simulink model "EMG_System"  (R2022a)
settings: Solver=FixedStepAuto  StartTime=0.0  StopTime=30  FixedStep=0.001  RelTol=1e-3
undefined symbols (not defined in the file): fdesignblkfcn, gcbh, Serial_Port, Standard_Devices
libraries: sldrtlib x4, dspxfrm3 x2, dspstat3 x2
settings Model: Creator=Damian  LastModifiedBy=lunde
settings ModelReferenceCC: EnableRefExpFcnMdlSchedulingChecks=off
settings RTWCC: Description=Generic Real-Time Target

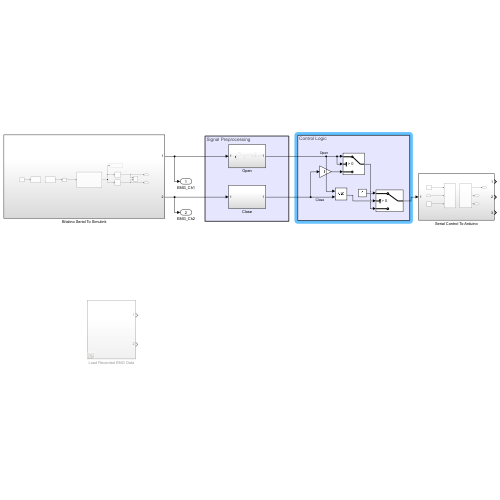
[thumbnail: Simulink's stored preview of the top-level diagram]
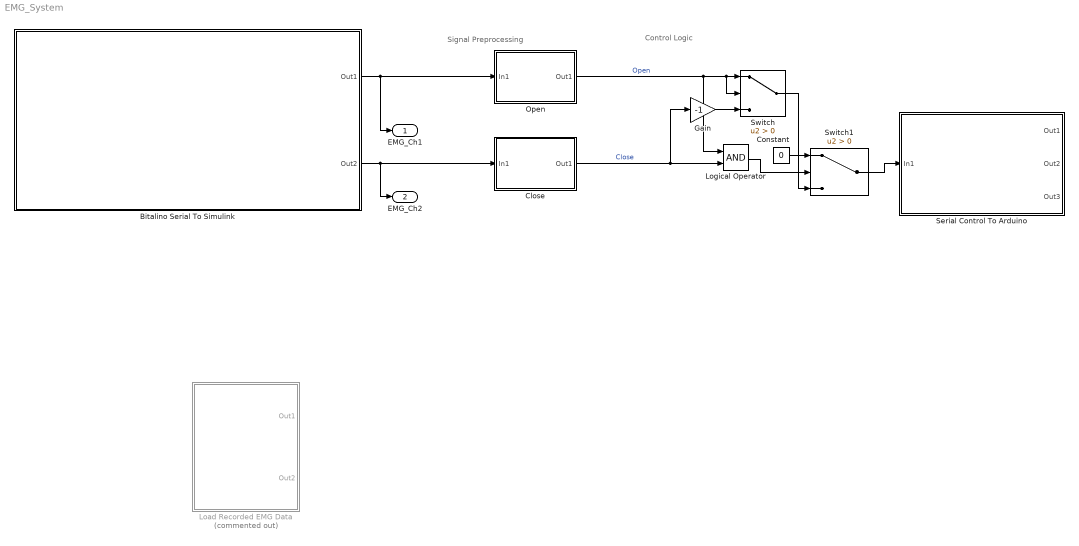
== system EMG_System ==
  note: Control Logic
  note: Signal Preprocessing
  Bitalino Serial To Simulink : Subsystem
  Close : Subsystem
  Constant : Constant  Value=0
  Gain : Gain  Gain=-1
  Load Recorded EMG Data : Subsystem  Commented=on
  Logical Operator : Logic  AllPortsSameDT=off  OutDataTypeStr=boolean
  Open : Subsystem
  Serial Control To Arduino : Subsystem
  Switch : Switch  Criteria=u2 > Threshold  SaturateOnIntegerOverflow=off  InputSameDT=off
  Switch1 : Switch  Criteria=u2 > Threshold  SaturateOnIntegerOverflow=off  InputSameDT=off
  EMG_Ch1 : Outport
  EMG_Ch2 : Outport  Port=2
  wires:
  Open/1(Out1) -> Switch/2, Switch/1, Logical Operator/1  "Open"
  Close/1(Out1) -> Logical Operator/2, Gain/1  "Close"
  Gain/1 -> Switch/3
  Logical Operator/1 -> Switch1/2
  Constant/1 -> Switch1/1
  Switch/1 -> Switch1/3
  Switch1/1 -> Serial Control To Arduino/1(In1)
  Bitalino Serial To Simulink/1(Out1) -> EMG_Ch1/1, Open/1(In1)
  Bitalino Serial To Simulink/2(Out2) -> EMG_Ch2/1, Close/1(In1)

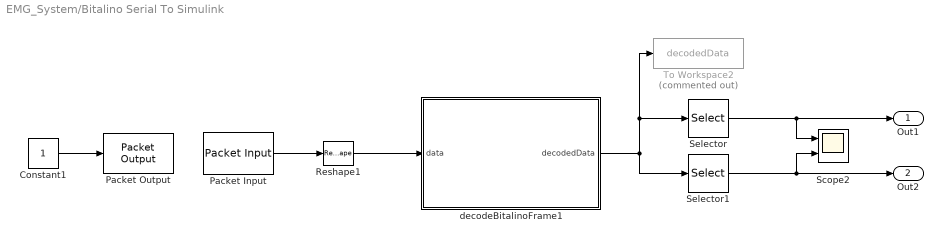
== system EMG_System/Bitalino Serial To Simulink ==
  Constant1 : Constant
  Packet Input : sldrtlib/Packet Input  SampleTime=0.001  MaxMissedTicks=10000  ShowMissedTicks=off  YieldWhenWaiting=on  DrvName=Standard_Devices/Serial_Port  DrvAddress=9  DrvOptions=[115200 8 0 0 0 0 0 0]  PacketSize=8  DataTypes='8*uint8'  ShowReady=off  ShowError=off  PacketID=1  ByteOrder=1  ShowTimestamp=off
      settings: AttributesFormatString=Serial Port [9]
  Packet Output : sldrtlib/Packet Output  SampleTime=0.001  MaxMissedTicks=10000  ShowMissedTicks=off  YieldWhenWaiting=on  DrvName=Standard_Devices/Serial_Port  DrvAddress=9  DrvOptions=[115200 8 0 0 0 0 0 0]  PacketSize=1  DataTypes='1*uint8'  ShowReady=off  ShowError=off  PacketID=1  ByteOrder=1  InitialValue=253  FinalValue=[]
      settings: AttributesFormatString=Serial Port [9]
  Reshape1 : Reshape  OutputDimensionality=Customize  OutputDimensions=[1,8]
  Scope2 : Scope  NumInputPorts=2
  Selector : Selector  InputPortWidth=2  IndexOptions=Index vector (dialog)  Indices=[1]  OutputSizes=1
  Selector1 : Selector  InputPortWidth=2  IndexOptions=Index vector (dialog)  Indices=[2]  OutputSizes=1
  To Workspace2 : ToWorkspace  Commented=on  VariableName=decodedData  SaveFormat=Timeseries  SampleTime=-1
  decodeBitalinoFrame1 : MATLAB Function  TreatAsAtomicUnit=on
  Out1 : Outport
  Out2 : Outport  Port=2
  wires:
  Selector/1 -> Out1/1, Scope2/1
  Selector1/1 -> Out2/1, Scope2/2
  Constant1/1 -> Packet Output/1
  Packet Input/1 -> Reshape1/1
  decodeBitalinoFrame1/1(decodedData) -> Selector1/1, To Workspace2/1, Selector/1
  Reshape1/1 -> decodeBitalinoFrame1/1(data)

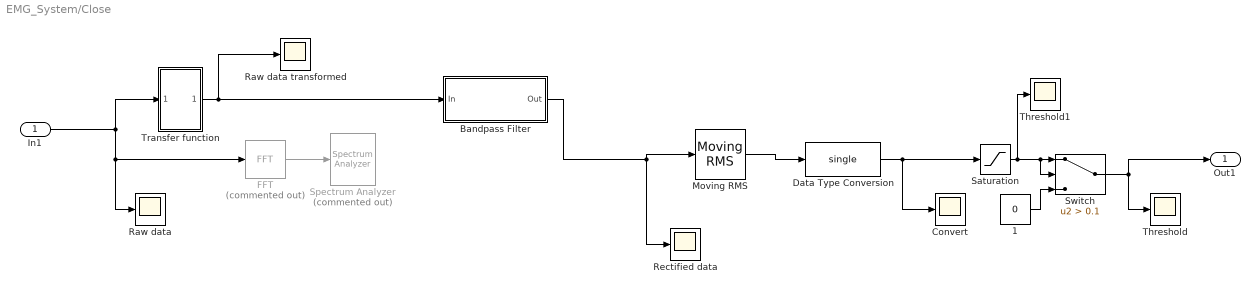
== system EMG_System/Close ==
  In1 : Inport
  1 : Constant  Value=0
  Bandpass Filter : Subsystem  DialogController=fdesignblkfcn  InitFcn=fdesignblkfcn(gcbh, {'InitFcn'});  mask(Bandpass Filter){}
      mask help: Design a bandpass filter
      settings: CopyFcn=fdesignblkfcn(gcbh, {'CopyFcn'});
      mask Help: helpview(mapfilelocation('dsp'), 'dspbandpassfilter');
      mask Display: disp('Bandpass');
  Convert : Scope
  Data Type Conversion : DataTypeConversion  OutMin=0  OutMax=1  OutDataTypeStr=single  RndMeth=Floor
  FFT : dspxfrm3/FFT  Commented=on  FFTImplementation=Auto  CompMethod=Table lookup  TableOpt=NEW  TableOptActive=Speed  BitRevOrder=off  Normalize=on  InheritFFTLength=on  FFTLength=64  WrapInput=on  roundingMode=Floor  overflowMode=off  firstCoeffDataTypeStr=Inherit: Same word length as input  firstCoeffLastDataTypeStr=Inherit: Same word length as input  outputMin=[]  outputMax=[]
  Moving RMS : dspstat3/Moving RMS  Method=Sliding window  ForgettingFactorPort=off  SpecifyWindowLength=on  WindowLength=100  ForgettingFactor=0.9  SimulateUsing=Code generation
      settings: SourceProductBaseCode=DS
  Raw data : Scope
  Raw data transformed : Scope
  Rectified data : Scope
  Saturation : Saturate  UpperLimit=0.8  LowerLimit=0.1
  Spectrum Analyzer : SpectrumAnalyzer  Commented=on
  Switch : Switch  Criteria=u2 > Threshold  Threshold=0.1  SaturateOnIntegerOverflow=off  InputSameDT=off
  Threshold : Scope
  Threshold1 : Scope
  Transfer function : Subsystem
  Out1 : Outport
  wires:
  Transfer function/1(Out1) -> Bandpass Filter/1(In), Raw data transformed/1
  FFT/1 -> Spectrum Analyzer/1
  1/1 -> Switch/3
  Bandpass Filter/1(Out) -> Moving RMS/1, Rectified data/1
  Moving RMS/1 -> Data Type Conversion/1
  Switch/1 -> Out1/1, Threshold/1
  In1/1 -> Transfer function/1(In1), Raw data/1, FFT/1
  Saturation/1 -> Threshold1/1, Switch/2, Switch/1
  Data Type Conversion/1 -> Saturation/1, Convert/1

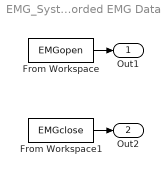
== system EMG_System/Load Recorded EMG Data ==
  From Workspace : FromWorkspace  VariableName=EMGopen
  From Workspace1 : FromWorkspace  VariableName=EMGclose
  Out1 : Outport
  Out2 : Outport  Port=2
  wires:
  From Workspace1/1 -> Out2/1
  From Workspace/1 -> Out1/1

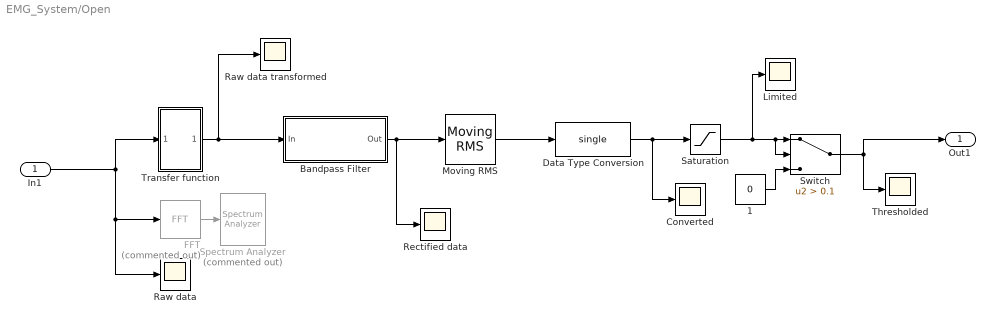
== system EMG_System/Open ==
  In1 : Inport
  1 : Constant  Value=0
  Bandpass Filter : Subsystem  DialogController=fdesignblkfcn  InitFcn=fdesignblkfcn(gcbh, {'InitFcn'});  mask(Bandpass Filter){}
      mask help: Design a bandpass filter
      settings: CopyFcn=fdesignblkfcn(gcbh, {'CopyFcn'});
      mask Help: helpview(mapfilelocation('dsp'), 'dspbandpassfilter');
      mask Display: disp('Bandpass');
  Converted : Scope
  Data Type Conversion : DataTypeConversion  OutMin=0  OutMax=1  OutDataTypeStr=single  RndMeth=Floor
  FFT : dspxfrm3/FFT  Commented=on  FFTImplementation=Auto  CompMethod=Table lookup  TableOpt=NEW  TableOptActive=Speed  BitRevOrder=off  Normalize=on  InheritFFTLength=on  FFTLength=64  WrapInput=on  roundingMode=Floor  overflowMode=off  firstCoeffDataTypeStr=Inherit: Same word length as input  firstCoeffLastDataTypeStr=Inherit: Same word length as input  outputMin=[]  outputMax=[]
  Limited : Scope
  Moving RMS : dspstat3/Moving RMS  Method=Sliding window  ForgettingFactorPort=off  SpecifyWindowLength=on  WindowLength=100  ForgettingFactor=0.9  SimulateUsing=Code generation
      settings: SourceProductBaseCode=DS
  Raw data : Scope
  Raw data transformed : Scope
  Rectified data : Scope
  Saturation : Saturate  UpperLimit=0.8  LowerLimit=0.1
  Spectrum Analyzer : SpectrumAnalyzer  Commented=on
  Switch : Switch  Criteria=u2 > Threshold  Threshold=0.1  SaturateOnIntegerOverflow=off  InputSameDT=off
  Thresholded : Scope
  Transfer function : Subsystem
  Out1 : Outport
  wires:
  Transfer function/1(Out1) -> Bandpass Filter/1(In), Raw data transformed/1
  FFT/1 -> Spectrum Analyzer/1
  1/1 -> Switch/3
  Bandpass Filter/1(Out) -> Moving RMS/1, Rectified data/1
  Moving RMS/1 -> Data Type Conversion/1
  Switch/1 -> Out1/1, Thresholded/1
  In1/1 -> Transfer function/1(In1), Raw data/1, FFT/1
  Saturation/1 -> Limited/1, Switch/2, Switch/1
  Data Type Conversion/1 -> Saturation/1, Converted/1

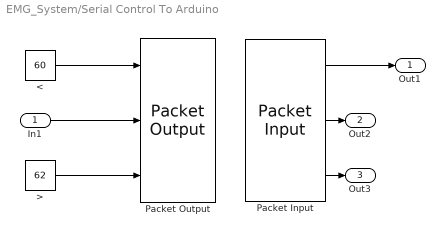
== system EMG_System/Serial Control To Arduino ==
  In1 : Inport  OutDataTypeStr=single  PortDimensions=1
  < : Constant  Value=60
  > : Constant  Value=62
  Packet Input : sldrtlib/Packet Input  SampleTime=0.1  MaxMissedTicks=1000  ShowMissedTicks=off  YieldWhenWaiting=off  DrvName=Standard_Devices/Serial_Port  DrvAddress=3  DrvOptions=[9600 8 0 0 0 0 0 0]  PacketSize=6  DataTypes={'1*single', '1*uint8', '1*uint8'}  ShowReady=off  ShowError=off  PacketID=1  ByteOrder=1  ShowTimestamp=off
      settings: AttributesFormatString=Serial Port [3]
  Packet Output : sldrtlib/Packet Output  SampleTime=0.1  MaxMissedTicks=1000  ShowMissedTicks=off  YieldWhenWaiting=off  DrvName=Standard_Devices/Serial_Port  DrvAddress=3  DrvOptions=[9600 8 0 0 0 0 0 0]  PacketSize=6  DataTypes={'1*uint8', '1*single', '1*uint8'}  ShowReady=off  ShowError=off  PacketID=1  ByteOrder=1  InitialValue=[]  FinalValue=[]
      settings: AttributesFormatString=Serial Port [3]
  Out1 : Outport
  Out2 : Outport  Port=2
  Out3 : Outport  Port=3
  wires:
  >/1 -> Packet Output/3
  In1/1 -> Packet Output/2
  </1 -> Packet Output/1
  Packet Input/2 -> Out2/1
  Packet Input/3 -> Out3/1
  Packet Input/1 -> Out1/1

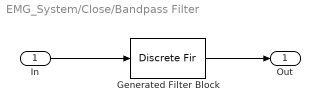
== system EMG_System/Close/Bandpass Filter ==
  In : Inport
  Generated Filter Block : DiscreteFir  Tag=BlockMethodSubSystem  Coefficients=[-0.000198473586190418182 0.00534852252952493484 0.0153234095334107579 0.0178570667191146684 0.00682248801041550508 -0.00274870515317482194 0.0030891279978422885 0.0111979036988692337 0.00456245530764537791 -0.0042151661328777134 0.00243546387977701222 0.00943183747086404935 -0.00146403536066665998 -0.011084600828395838 -0.00059029452559431156 0.00547540465791776249 -0.0119371461871073409 -0.0215599836706455474 -0.00473015163609309848 -0.000830348429932785187 -0.0270963317844445002 -0.034209054098530034 -0.00755561394207852031 -0.00849262478015036168 -0.0471568823138692056 -0.0469015880042323238 -0.00421271941163124924 -0.0158506365642964719 -0.0755462338263607064 -0.0571919323183570777 0.0195397096648971362 -0.0211950204421756522 -0.145410009473957602 -0.0629799708976308825 0.274125237654004761 0.476886321904536448 0.274125237654004761 -0.0629799708976308825 -0.145410009473957602 -0.0211950204421756522 0.0195397096648971362 -0.0571919323183570777 -0.0755462338263607064 -0.0158506365642964719 -0.00421271941163124924 -0.0469015880042323238 -0.0471568823138692056 -0.00849262478015036168 -0.00755561394207852031 -0.034209054098530034 -0.0270963317844445002 -0.000830348429932785187 -0.00473015163609309848 -0.0215599836706455474 -0.0119371461871073409 0.00547540465791776249 -0.00059029452559431156 -0.011084600828395838 -0.00146403536066665998 0.00943183747086404935 0.00243546387977701222 -0.0042151661328777134 0.00456245530764537791 0.0111979036988692337 0.0030891279978422885 -0.00274870515317482194 0.00682248801041550508 0.0178570667191146684 0.0153234095334107579 0.00534852252952493484 -0.000198473586190418182]  InputProcessing=Columns as channels (frame based)
  Out : Outport  VectorParamsAs1DForOutWhenUnconnected=off
  wires:
  In/1 -> Generated Filter Block/1
  Generated Filter Block/1 -> Out/1

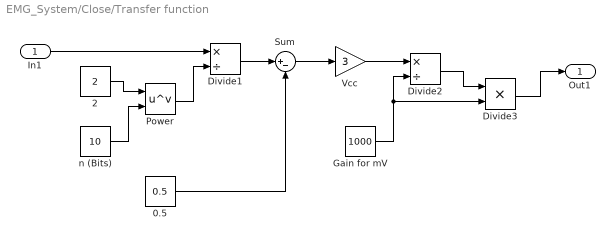
== system EMG_System/Close/Transfer function ==
  In1 : Inport
  0.5 : Constant  Value=0.5
  2 : Constant  Value=2
  Divide1 : Product  Inputs=*/
  Divide2 : Product  Inputs=*/
  Divide3 : Product  Inputs=**
  Gain for mV : Constant  Value=1000
  Power : Math  Operator=pow
  Sum : Sum  Inputs=|+-
  Vcc : Gain  Gain=3
  n (Bits) : Constant  Value=10
  Out1 : Outport
  wires:
  n (Bits)/1 -> Power/2
  In1/1 -> Divide1/1
  0.5/1 -> Sum/2
  Gain for mV/1 -> Divide3/2, Divide2/2
  Vcc/1 -> Divide2/1
  2/1 -> Power/1
  Power/1 -> Divide1/2
  Divide2/1 -> Divide3/1
  Divide3/1 -> Out1/1
  Divide1/1 -> Sum/1
  Sum/1 -> Vcc/1

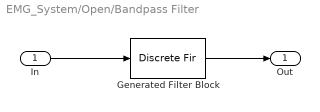
== system EMG_System/Open/Bandpass Filter ==
  In : Inport
  Generated Filter Block : DiscreteFir  Tag=BlockMethodSubSystem  Coefficients=[-0.000198473586190418182 0.00534852252952493484 0.0153234095334107579 0.0178570667191146684 0.00682248801041550508 -0.00274870515317482194 0.0030891279978422885 0.0111979036988692337 0.00456245530764537791 -0.0042151661328777134 0.00243546387977701222 0.00943183747086404935 -0.00146403536066665998 -0.011084600828395838 -0.00059029452559431156 0.00547540465791776249 -0.0119371461871073409 -0.0215599836706455474 -0.00473015163609309848 -0.000830348429932785187 -0.0270963317844445002 -0.034209054098530034 -0.00755561394207852031 -0.00849262478015036168 -0.0471568823138692056 -0.0469015880042323238 -0.00421271941163124924 -0.0158506365642964719 -0.0755462338263607064 -0.0571919323183570777 0.0195397096648971362 -0.0211950204421756522 -0.145410009473957602 -0.0629799708976308825 0.274125237654004761 0.476886321904536448 0.274125237654004761 -0.0629799708976308825 -0.145410009473957602 -0.0211950204421756522 0.0195397096648971362 -0.0571919323183570777 -0.0755462338263607064 -0.0158506365642964719 -0.00421271941163124924 -0.0469015880042323238 -0.0471568823138692056 -0.00849262478015036168 -0.00755561394207852031 -0.034209054098530034 -0.0270963317844445002 -0.000830348429932785187 -0.00473015163609309848 -0.0215599836706455474 -0.0119371461871073409 0.00547540465791776249 -0.00059029452559431156 -0.011084600828395838 -0.00146403536066665998 0.00943183747086404935 0.00243546387977701222 -0.0042151661328777134 0.00456245530764537791 0.0111979036988692337 0.0030891279978422885 -0.00274870515317482194 0.00682248801041550508 0.0178570667191146684 0.0153234095334107579 0.00534852252952493484 -0.000198473586190418182]  InputProcessing=Columns as channels (frame based)
  Out : Outport  VectorParamsAs1DForOutWhenUnconnected=off
  wires:
  In/1 -> Generated Filter Block/1
  Generated Filter Block/1 -> Out/1

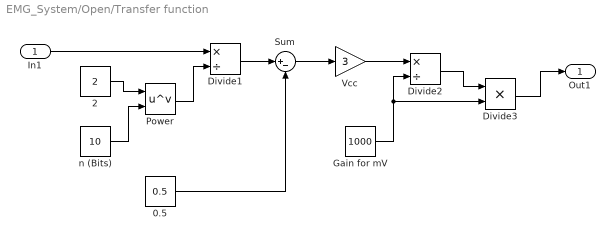
== system EMG_System/Open/Transfer function ==
  In1 : Inport
  0.5 : Constant  Value=0.5
  2 : Constant  Value=2
  Divide1 : Product  Inputs=*/
  Divide2 : Product  Inputs=*/
  Divide3 : Product  Inputs=**
  Gain for mV : Constant  Value=1000
  Power : Math  Operator=pow
  Sum : Sum  Inputs=|+-
  Vcc : Gain  Gain=3
  n (Bits) : Constant  Value=10
  Out1 : Outport
  wires:
  n (Bits)/1 -> Power/2
  In1/1 -> Divide1/1
  0.5/1 -> Sum/2
  Gain for mV/1 -> Divide3/2, Divide2/2
  Vcc/1 -> Divide2/1
  2/1 -> Power/1
  Power/1 -> Divide1/2
  Divide2/1 -> Divide3/1
  Divide3/1 -> Out1/1
  Divide1/1 -> Sum/1
  Sum/1 -> Vcc/1

== matlab function EMG_System/Bitalino Serial To Simulink/decodeBitalinoFrame1 ==
  data: data input uint8; decodedData output
function decodedData = decodeBitalinoFrame(data)
% Decode a single frame of data
% Decode the data Frames and return an array of data
% NOTE: The following code does bitwise operations to decode the
% data in each packet. Refer to the Bitalino's MCU block
% datasheet for information on ordering of data within a packet
% http://bitalino.com/datasheets/MCU_Block_Datasheet.pdf

% Define variables
% Output data: [packetNumber D0 D1 D2 D3 A0 A1 A2 A3 A4 A5];

decodedData = zeros(1,2);
for i = 1:size(data,1)
    % Only decode CRC if the hidden property, VerifyCRC, is
    % true. NOTE: Doing this has a significant performance
    % impact.
    if (1) % obj.VerifyCRC
        % Extract CRC
        CRC = bitand(data(i,8), 15,'uint8');                         % 15 = bin2dec('00001111')
        data(i,8) = bitand(data(i,8),240,'uint8');                  % 240 = bin2dec('11110000')
        % Decode the Cyclic Redundancy Check and cross verify
        data(i,8) = bitand(data(i,8),240);
        calcCRC = uint8(0);
        for j = 1:1:8
            for bit = 7:-1:0
                calcCRC = bitshift(calcCRC,1,'uint8');
                if bitand(calcCRC,16)
                    calcCRC = bitxor(calcCRC,3,'uint8');
                end
                calcCRC = bitxor(calcCRC, ...
                    bitand(1, bitshift(data(i,j),-1*bit)),'uint8');
            end
        end
        calcCRC = bitand(uint8(calcCRC),15,'uint8');
        if ~isequal(CRC,calcCRC)
            %throw(MException('bitalino:read:CRCError',sprintf('Error when decoding frame. CRC = %u, calculated CRC = %u',CRC, calcCRC)));
        end
    end
    
    % Decode the Sequential Number (packetNumber). This ranges from 0-15
    packetNumber = bitshift(data(i,8),-4,'uint8');
    
    % Decode digitalInputs
    D0 = bitshift(bitand(data(i,7),128),-7);                % 128 = bin2dec('10000000');
    D1 = bitshift(bitand(data(i,7),64),-6);                 % 64 = bin2dec('01000000');
    D2 = bitshift(bitand(data(i,7),32),-5);                 % 32 = bin2dec('00100000');
    D3 = bitshift(bitand(data(i,7),16),-4);                 % 16 = bin2dec('00010000');

    % Decode A0 bits. This should have a range of 0-1023
    A0 = bitor(bitshift(cast(bitand(data(i,7),15,'uint8'),'uint16'),6,'uint16'), ...
        cast(bitshift(data(i,6),-2,'uint8'),'uint16'), 'uint16');
    
    % Decode A1 bits. This should have a range of 0-1023
    A1 = bitor(bitshift(cast(bitand(data(i,6),3,'uint8'),'uint16'),-8,'uint16'), ...
        cast(data(i,5),'uint16'));
    
    % Decode A2 bits. This should have a range of 0-1023
    A2 = bitor(bitshift(cast(data(i,4),'uint16'),2,'uint16'), ...
        cast(bitshift(data(i,3),-6,'uint8'),'uint16'));
    
    % Decode A3 bits. This should have a range of 0-1023
    A3 = bitor(bitshift(cast(bitand(data(i,3),63,'uint8'),'uint16'),4,'uint16'), ...
        cast(bitshift(data(i,2),-4,'uint8'),'uint16'));
    
    % Decode A4 bits. This has a range of 0-63
    A4 = bitor(bitshift(bitand(data(i,2),15,'uint8'),2,'uint8'), ...
        bitshift(data(i,1),-6),'uint8');
    
    % Decode A5 bits. This has a range of 0-63
    A5 = bitand(data(i,1),63,'uint8');
    
    decodedData(i,:) = [A0 A2]; %[packetNumber D0 D1 D2 D3 A0 A1 A2 A3 A4 A5];
end
